simulink model "phantomx_sim_zero"  (R2025b)
settings: Solver=daessc  StartTime=0.0  StopTime=20  RelTol=1e-3
InitFcn:
  | % Parametri del filtro
  | num_filters = 18;       % Numero di filtri in parallelo (i tuoi 18 giunti/segnali)
  | tau = 0.05;             % Costante di tempo del filtro in secondi (modificabile)
  | a = 1 / tau;            % Polo del sistema
  | 
  | % 1. Creazione delle Matrici di Stato (State-Space)
  | % Matrice A (Dinamica del sistema): Diagonale con i poli
  | A = -a * eye(num_filters);
  | 
  | % Matrice B (Matrice di ingresso): Diagonale per mappare ogni input al suo stato
  | B = a * eye(num_filters);
  | 
  | % Matrice C (Matrice di uscita): Identità (vogliamo leggere gli stati direttamente)
  | C = eye(num_filters);
  | 
  | % Matrice D (Feedforward): Matrice di zeri (nessun collegamento diretto input-output)
  | D = zeros(num_filters, num_filters);
  | 
  | % 2. Creazione dell'oggetto State-Space in MATLAB
  | sys_filter = ss(A, B, C, D);
  | 
  | % Aggiungiamo i nomi per tenere tutto in ordine (opzionale ma consigliato)
  | sys_filter.InputName = strcat('Action_In_', string(1:num_filters));
  | sys_filter.OutputName = strcat('Filtered_Action_Out_', string(1:num_filters));
  | sys_filter.StateName = strcat('State_', string(1:num_filters));
  | 
  | % Mostra le proprietà del sistema creato
  | disp('Sistema State-Space creato con successo:');
  | sys_filter
  | 
  | run init_gait.m
undefined symbols (not defined in the file or in its folder): gait, X, Y, Z
libraries: sm_lib x298, nesl_utility x94, robotmaniplib x1
(part 5 of 5)

== system phantomx_sim_zero/tibia_lr ==
  Inertia : sm_lib/Body Elements/Inertia  InertiaType=Custom  Mass=0.024357719  MassUnits=kg  CenterOfMass=[0, 0, 0]  CenterOfMassUnits=m  MomentsOfInertia=[0.0051411124, 0.0081915737, 0.0011379812]  MomentsOfInertiaUnits=kg*m^2  ProductsOfInertia=[-1.9223094e-05, -2.4729049e-05, -0.0005753025500000001]  ProductsOfInertiaUnits=kg*m^2  GraphicType=None  MarkerShape=Inertia  MarkerSize=20  GraphicVisPropType=SimpleVisualProperties  GraphicDiffuseColor=[0.5 0.5 0.5]  GraphicOpacity=1  GraphicSpecularColor=[0.5 0.5 0.5 1.0]  GraphicAmbientColor=[0.15 0.15 0.15 1.0]  GraphicEmissiveColor=[0.0 0.0 0.0 1.0]  GraphicShininess=75
  InertiaOriginTransform : sm_lib/Frames and Transforms/Rigid Transform  RotationMethod=RotationSequence  FollAlignAxisA=+X  BaseAlignAxisA=+Y  FollAlignAxisB=+Y  BaseAlignAxisB=+Z  RotationStandardAxis=+Z  RotationAngle=0  RotationAngleUnits=deg  RotationArbitraryAxis=[0 0 1]  RotationSequenceAxes=BaseAxes  RotationSequence=XYZ  RotationSequenceAngles=[0, 0, 0]  RotationSequenceAnglesUnits=rad  RotationMatrix=[1 0 0;0 1 0;0 0 1]  Quaternion=[1 0 0 0]  TranslationMethod=Cartesian  TranslationCartesianOffset=[0, 0, 0]  TranslationCartesianOffsetUnits=m  TranslationStandardAxis=+Z  TranslationStandardOffset=0  TranslationStandardOffsetUnits=m  TranslationROffset=0  TranslationROffsetUnits=m  TranslationThetaOffset=0  TranslationThetaOffsetUnits=deg  TranslationZOffset=0  TranslationZOffsetUnits=m
  ReferenceFrame : sm_lib/Frames and Transforms/Reference Frame
  Visual : sm_lib/Body Elements/File Solid  ExtGeomFileName=phantomx_description-master/meshes/tibia_l.STL  UnitType=Custom  ExtGeomFileUnits=m  StepReaderType=HEX  ExportConvexHullGeometry=off  InertiaType=Custom  BasedOnType=DensityFromFile  Density=1000  DensityUnits=kg/m^3  Mass=0  MassUnits=kg  CenterOfMass=[0, 0, 0]  CenterOfMassUnits=m  MomentsOfInertia=[0, 0, 0]  MomentsOfInertiaUnits=kg*m^2  ProductsOfInertia=[0, 0, 0]  ProductsOfInertiaUnits=kg*m^2  GraphicType=FromGeometry  MarkerShape=Sphere  MarkerSize=10  GraphicVisPropType=SimpleVisualProperties  GraphicDiffuseColor=[0.2, 0.2, 0.2]  GraphicOpacity=1  GraphicSpecularColor=[0.5 0.5 0.5 1.0]  GraphicAmbientColor=[0.15 0.15 0.15 1.0]  GraphicEmissiveColor=[0.0 0.0 0.0 1.0]  GraphicShininess=75  DoExposeReferenceFrame=on  SerializedFrames=<Frames/>
  VisualOriginTransform : sm_lib/Frames and Transforms/Rigid Transform  RotationMethod=RotationSequence  FollAlignAxisA=+X  BaseAlignAxisA=+Y  FollAlignAxisB=+Y  BaseAlignAxisB=+Z  RotationStandardAxis=+Z  RotationAngle=0  RotationAngleUnits=deg  RotationArbitraryAxis=[0 0 1]  RotationSequenceAxes=BaseAxes  RotationSequence=XYZ  RotationSequenceAngles=[0, 0, 0]  RotationSequenceAnglesUnits=rad  RotationMatrix=[1 0 0;0 1 0;0 0 1]  Quaternion=[1 0 0 0]  TranslationMethod=Cartesian  TranslationCartesianOffset=[0, 0, 0]  TranslationCartesianOffsetUnits=m  TranslationStandardAxis=+Z  TranslationStandardOffset=0  TranslationStandardOffsetUnits=m  TranslationROffset=0  TranslationROffsetUnits=m  TranslationThetaOffset=0  TranslationThetaOffsetUnits=deg  TranslationZOffset=0  TranslationZOffsetUnits=m
  j_tibia_lr_AxisInvTransform : sm_lib/Frames and Transforms/Rigid Transform  RotationMethod=ArbitraryAxis  FollAlignAxisA=+X  BaseAlignAxisA=+Y  FollAlignAxisB=+Y  BaseAlignAxisB=+Z  RotationStandardAxis=+Z  RotationAngle=1.570796326794897  RotationAngleUnits=rad  RotationArbitraryAxis=[-0, 1, 0]  RotationSequenceAxes=FollowerAxes  RotationSequence=XYX  RotationSequenceAngles=[0 0 0]  RotationSequenceAnglesUnits=deg  RotationMatrix=[1 0 0;0 1 0;0 0 1]  Quaternion=[1 0 0 0]  TranslationMethod=Cartesian  TranslationCartesianOffset=[0, 0, 0]  TranslationCartesianOffsetUnits=m  TranslationStandardAxis=+Z  TranslationStandardOffset=0  TranslationStandardOffsetUnits=m  TranslationROffset=0  TranslationROffsetUnits=m  TranslationThetaOffset=0  TranslationThetaOffsetUnits=deg  TranslationZOffset=0  TranslationZOffsetUnits=m
  F : PMIOPort  Side=Left
  connections:
  Inertia/RConn1 -- InertiaOriginTransform/RConn1
  ReferenceFrame/RConn1 -- InertiaOriginTransform/LConn1 -- VisualOriginTransform/LConn1 -- j_tibia_lr_AxisInvTransform/LConn1
  Visual/RConn1 -- VisualOriginTransform/RConn1
  j_tibia_lr_AxisInvTransform/RConn1 -- F/RConn1

== system phantomx_sim_zero/tibia_rf ==
  Inertia : sm_lib/Body Elements/Inertia  InertiaType=Custom  Mass=0.024357719  MassUnits=kg  CenterOfMass=[0, 0, 0]  CenterOfMassUnits=m  MomentsOfInertia=[0.0051411124, 0.0081915737, 0.0011379812]  MomentsOfInertiaUnits=kg*m^2  ProductsOfInertia=[-1.9223094e-05, -2.4729049e-05, -0.0005753025500000001]  ProductsOfInertiaUnits=kg*m^2  GraphicType=None  MarkerShape=Inertia  MarkerSize=20  GraphicVisPropType=SimpleVisualProperties  GraphicDiffuseColor=[0.5 0.5 0.5]  GraphicOpacity=1  GraphicSpecularColor=[0.5 0.5 0.5 1.0]  GraphicAmbientColor=[0.15 0.15 0.15 1.0]  GraphicEmissiveColor=[0.0 0.0 0.0 1.0]  GraphicShininess=75
  InertiaOriginTransform : sm_lib/Frames and Transforms/Rigid Transform  RotationMethod=RotationSequence  FollAlignAxisA=+X  BaseAlignAxisA=+Y  FollAlignAxisB=+Y  BaseAlignAxisB=+Z  RotationStandardAxis=+Z  RotationAngle=0  RotationAngleUnits=deg  RotationArbitraryAxis=[0 0 1]  RotationSequenceAxes=BaseAxes  RotationSequence=XYZ  RotationSequenceAngles=[0, 0, 0]  RotationSequenceAnglesUnits=rad  RotationMatrix=[1 0 0;0 1 0;0 0 1]  Quaternion=[1 0 0 0]  TranslationMethod=Cartesian  TranslationCartesianOffset=[0, 0, 0]  TranslationCartesianOffsetUnits=m  TranslationStandardAxis=+Z  TranslationStandardOffset=0  TranslationStandardOffsetUnits=m  TranslationROffset=0  TranslationROffsetUnits=m  TranslationThetaOffset=0  TranslationThetaOffsetUnits=deg  TranslationZOffset=0  TranslationZOffsetUnits=m
  ReferenceFrame : sm_lib/Frames and Transforms/Reference Frame
  Visual : sm_lib/Body Elements/File Solid  ExtGeomFileName=phantomx_description-master/meshes/tibia_l.STL  UnitType=Custom  ExtGeomFileUnits=m  StepReaderType=HEX  ExportConvexHullGeometry=off  InertiaType=Custom  BasedOnType=DensityFromFile  Density=1000  DensityUnits=kg/m^3  Mass=0  MassUnits=kg  CenterOfMass=[0, 0, 0]  CenterOfMassUnits=m  MomentsOfInertia=[0, 0, 0]  MomentsOfInertiaUnits=kg*m^2  ProductsOfInertia=[0, 0, 0]  ProductsOfInertiaUnits=kg*m^2  GraphicType=FromGeometry  MarkerShape=Sphere  MarkerSize=10  GraphicVisPropType=SimpleVisualProperties  GraphicDiffuseColor=[0.2, 0.2, 0.2]  GraphicOpacity=1  GraphicSpecularColor=[0.5 0.5 0.5 1.0]  GraphicAmbientColor=[0.15 0.15 0.15 1.0]  GraphicEmissiveColor=[0.0 0.0 0.0 1.0]  GraphicShininess=75  DoExposeReferenceFrame=on  SerializedFrames=<Frames/>
  VisualOriginTransform : sm_lib/Frames and Transforms/Rigid Transform  RotationMethod=RotationSequence  FollAlignAxisA=+X  BaseAlignAxisA=+Y  FollAlignAxisB=+Y  BaseAlignAxisB=+Z  RotationStandardAxis=+Z  RotationAngle=0  RotationAngleUnits=deg  RotationArbitraryAxis=[0 0 1]  RotationSequenceAxes=BaseAxes  RotationSequence=XYZ  RotationSequenceAngles=[0, 0, 0]  RotationSequenceAnglesUnits=rad  RotationMatrix=[1 0 0;0 1 0;0 0 1]  Quaternion=[1 0 0 0]  TranslationMethod=Cartesian  TranslationCartesianOffset=[0, 0, 0]  TranslationCartesianOffsetUnits=m  TranslationStandardAxis=+Z  TranslationStandardOffset=0  TranslationStandardOffsetUnits=m  TranslationROffset=0  TranslationROffsetUnits=m  TranslationThetaOffset=0  TranslationThetaOffsetUnits=deg  TranslationZOffset=0  TranslationZOffsetUnits=m
  j_tibia_rf_AxisInvTransform : sm_lib/Frames and Transforms/Rigid Transform  RotationMethod=ArbitraryAxis  FollAlignAxisA=+X  BaseAlignAxisA=+Y  FollAlignAxisB=+Y  BaseAlignAxisB=+Z  RotationStandardAxis=+Z  RotationAngle=1.570796326794897  RotationAngleUnits=rad  RotationArbitraryAxis=[-0, 1, 0]  RotationSequenceAxes=FollowerAxes  RotationSequence=XYX  RotationSequenceAngles=[0 0 0]  RotationSequenceAnglesUnits=deg  RotationMatrix=[1 0 0;0 1 0;0 0 1]  Quaternion=[1 0 0 0]  TranslationMethod=Cartesian  TranslationCartesianOffset=[0, 0, 0]  TranslationCartesianOffsetUnits=m  TranslationStandardAxis=+Z  TranslationStandardOffset=0  TranslationStandardOffsetUnits=m  TranslationROffset=0  TranslationROffsetUnits=m  TranslationThetaOffset=0  TranslationThetaOffsetUnits=deg  TranslationZOffset=0  TranslationZOffsetUnits=m
  F : PMIOPort  Side=Left
  connections:
  Inertia/RConn1 -- InertiaOriginTransform/RConn1
  ReferenceFrame/RConn1 -- InertiaOriginTransform/LConn1 -- VisualOriginTransform/LConn1 -- j_tibia_rf_AxisInvTransform/LConn1
  Visual/RConn1 -- VisualOriginTransform/RConn1
  j_tibia_rf_AxisInvTransform/RConn1 -- F/RConn1

== system phantomx_sim_zero/tibia_rm ==
  Inertia : sm_lib/Body Elements/Inertia  InertiaType=Custom  Mass=0.024357719  MassUnits=kg  CenterOfMass=[0, 0, 0]  CenterOfMassUnits=m  MomentsOfInertia=[0.0051411124, 0.0081915737, 0.0011379812]  MomentsOfInertiaUnits=kg*m^2  ProductsOfInertia=[-1.9223094e-05, -2.4729049e-05, -0.0005753025500000001]  ProductsOfInertiaUnits=kg*m^2  GraphicType=None  MarkerShape=Inertia  MarkerSize=20  GraphicVisPropType=SimpleVisualProperties  GraphicDiffuseColor=[0.5 0.5 0.5]  GraphicOpacity=1  GraphicSpecularColor=[0.5 0.5 0.5 1.0]  GraphicAmbientColor=[0.15 0.15 0.15 1.0]  GraphicEmissiveColor=[0.0 0.0 0.0 1.0]  GraphicShininess=75
  InertiaOriginTransform : sm_lib/Frames and Transforms/Rigid Transform  RotationMethod=RotationSequence  FollAlignAxisA=+X  BaseAlignAxisA=+Y  FollAlignAxisB=+Y  BaseAlignAxisB=+Z  RotationStandardAxis=+Z  RotationAngle=0  RotationAngleUnits=deg  RotationArbitraryAxis=[0 0 1]  RotationSequenceAxes=BaseAxes  RotationSequence=XYZ  RotationSequenceAngles=[0, 0, 0]  RotationSequenceAnglesUnits=rad  RotationMatrix=[1 0 0;0 1 0;0 0 1]  Quaternion=[1 0 0 0]  TranslationMethod=Cartesian  TranslationCartesianOffset=[0, 0, 0]  TranslationCartesianOffsetUnits=m  TranslationStandardAxis=+Z  TranslationStandardOffset=0  TranslationStandardOffsetUnits=m  TranslationROffset=0  TranslationROffsetUnits=m  TranslationThetaOffset=0  TranslationThetaOffsetUnits=deg  TranslationZOffset=0  TranslationZOffsetUnits=m
  ReferenceFrame : sm_lib/Frames and Transforms/Reference Frame
  Visual : sm_lib/Body Elements/File Solid  ExtGeomFileName=phantomx_description-master/meshes/tibia_l.STL  UnitType=Custom  ExtGeomFileUnits=m  StepReaderType=HEX  ExportConvexHullGeometry=off  InertiaType=Custom  BasedOnType=DensityFromFile  Density=1000  DensityUnits=kg/m^3  Mass=0  MassUnits=kg  CenterOfMass=[0, 0, 0]  CenterOfMassUnits=m  MomentsOfInertia=[0, 0, 0]  MomentsOfInertiaUnits=kg*m^2  ProductsOfInertia=[0, 0, 0]  ProductsOfInertiaUnits=kg*m^2  GraphicType=FromGeometry  MarkerShape=Sphere  MarkerSize=10  GraphicVisPropType=SimpleVisualProperties  GraphicDiffuseColor=[0.2, 0.2, 0.2]  GraphicOpacity=1  GraphicSpecularColor=[0.5 0.5 0.5 1.0]  GraphicAmbientColor=[0.15 0.15 0.15 1.0]  GraphicEmissiveColor=[0.0 0.0 0.0 1.0]  GraphicShininess=75  DoExposeReferenceFrame=on  SerializedFrames=<Frames/>
  VisualOriginTransform : sm_lib/Frames and Transforms/Rigid Transform  RotationMethod=RotationSequence  FollAlignAxisA=+X  BaseAlignAxisA=+Y  FollAlignAxisB=+Y  BaseAlignAxisB=+Z  RotationStandardAxis=+Z  RotationAngle=0  RotationAngleUnits=deg  RotationArbitraryAxis=[0 0 1]  RotationSequenceAxes=BaseAxes  RotationSequence=XYZ  RotationSequenceAngles=[0, 0, 0]  RotationSequenceAnglesUnits=rad  RotationMatrix=[1 0 0;0 1 0;0 0 1]  Quaternion=[1 0 0 0]  TranslationMethod=Cartesian  TranslationCartesianOffset=[0, 0, 0]  TranslationCartesianOffsetUnits=m  TranslationStandardAxis=+Z  TranslationStandardOffset=0  TranslationStandardOffsetUnits=m  TranslationROffset=0  TranslationROffsetUnits=m  TranslationThetaOffset=0  TranslationThetaOffsetUnits=deg  TranslationZOffset=0  TranslationZOffsetUnits=m
  j_tibia_rm_AxisInvTransform : sm_lib/Frames and Transforms/Rigid Transform  RotationMethod=ArbitraryAxis  FollAlignAxisA=+X  BaseAlignAxisA=+Y  FollAlignAxisB=+Y  BaseAlignAxisB=+Z  RotationStandardAxis=+Z  RotationAngle=1.570796326794897  RotationAngleUnits=rad  RotationArbitraryAxis=[-0, 1, 0]  RotationSequenceAxes=FollowerAxes  RotationSequence=XYX  RotationSequenceAngles=[0 0 0]  RotationSequenceAnglesUnits=deg  RotationMatrix=[1 0 0;0 1 0;0 0 1]  Quaternion=[1 0 0 0]  TranslationMethod=Cartesian  TranslationCartesianOffset=[0, 0, 0]  TranslationCartesianOffsetUnits=m  TranslationStandardAxis=+Z  TranslationStandardOffset=0  TranslationStandardOffsetUnits=m  TranslationROffset=0  TranslationROffsetUnits=m  TranslationThetaOffset=0  TranslationThetaOffsetUnits=deg  TranslationZOffset=0  TranslationZOffsetUnits=m
  F : PMIOPort  Side=Left
  connections:
  Inertia/RConn1 -- InertiaOriginTransform/RConn1
  ReferenceFrame/RConn1 -- InertiaOriginTransform/LConn1 -- VisualOriginTransform/LConn1 -- j_tibia_rm_AxisInvTransform/LConn1
  Visual/RConn1 -- VisualOriginTransform/RConn1
  j_tibia_rm_AxisInvTransform/RConn1 -- F/RConn1

== system phantomx_sim_zero/tibia_rr ==
  Inertia : sm_lib/Body Elements/Inertia  InertiaType=Custom  Mass=0.024357719  MassUnits=kg  CenterOfMass=[0, 0, 0]  CenterOfMassUnits=m  MomentsOfInertia=[0.0051411124, 0.0081915737, 0.0011379812]  MomentsOfInertiaUnits=kg*m^2  ProductsOfInertia=[-1.9223094e-05, -2.4729049e-05, -0.0005753025500000001]  ProductsOfInertiaUnits=kg*m^2  GraphicType=None  MarkerShape=Inertia  MarkerSize=20  GraphicVisPropType=SimpleVisualProperties  GraphicDiffuseColor=[0.5 0.5 0.5]  GraphicOpacity=1  GraphicSpecularColor=[0.5 0.5 0.5 1.0]  GraphicAmbientColor=[0.15 0.15 0.15 1.0]  GraphicEmissiveColor=[0.0 0.0 0.0 1.0]  GraphicShininess=75
  InertiaOriginTransform : sm_lib/Frames and Transforms/Rigid Transform  RotationMethod=RotationSequence  FollAlignAxisA=+X  BaseAlignAxisA=+Y  FollAlignAxisB=+Y  BaseAlignAxisB=+Z  RotationStandardAxis=+Z  RotationAngle=0  RotationAngleUnits=deg  RotationArbitraryAxis=[0 0 1]  RotationSequenceAxes=BaseAxes  RotationSequence=XYZ  RotationSequenceAngles=[0, 0, 0]  RotationSequenceAnglesUnits=rad  RotationMatrix=[1 0 0;0 1 0;0 0 1]  Quaternion=[1 0 0 0]  TranslationMethod=Cartesian  TranslationCartesianOffset=[0, 0, 0]  TranslationCartesianOffsetUnits=m  TranslationStandardAxis=+Z  TranslationStandardOffset=0  TranslationStandardOffsetUnits=m  TranslationROffset=0  TranslationROffsetUnits=m  TranslationThetaOffset=0  TranslationThetaOffsetUnits=deg  TranslationZOffset=0  TranslationZOffsetUnits=m
  ReferenceFrame : sm_lib/Frames and Transforms/Reference Frame
  Visual : sm_lib/Body Elements/File Solid  ExtGeomFileName=phantomx_description-master/meshes/tibia_l.STL  UnitType=Custom  ExtGeomFileUnits=m  StepReaderType=HEX  ExportConvexHullGeometry=off  InertiaType=Custom  BasedOnType=DensityFromFile  Density=1000  DensityUnits=kg/m^3  Mass=0  MassUnits=kg  CenterOfMass=[0, 0, 0]  CenterOfMassUnits=m  MomentsOfInertia=[0, 0, 0]  MomentsOfInertiaUnits=kg*m^2  ProductsOfInertia=[0, 0, 0]  ProductsOfInertiaUnits=kg*m^2  GraphicType=FromGeometry  MarkerShape=Sphere  MarkerSize=10  GraphicVisPropType=SimpleVisualProperties  GraphicDiffuseColor=[0.2, 0.2, 0.2]  GraphicOpacity=1  GraphicSpecularColor=[0.5 0.5 0.5 1.0]  GraphicAmbientColor=[0.15 0.15 0.15 1.0]  GraphicEmissiveColor=[0.0 0.0 0.0 1.0]  GraphicShininess=75  DoExposeReferenceFrame=on  SerializedFrames=<Frames/>
  VisualOriginTransform : sm_lib/Frames and Transforms/Rigid Transform  RotationMethod=RotationSequence  FollAlignAxisA=+X  BaseAlignAxisA=+Y  FollAlignAxisB=+Y  BaseAlignAxisB=+Z  RotationStandardAxis=+Z  RotationAngle=0  RotationAngleUnits=deg  RotationArbitraryAxis=[0 0 1]  RotationSequenceAxes=BaseAxes  RotationSequence=XYZ  RotationSequenceAngles=[0, 0, 0]  RotationSequenceAnglesUnits=rad  RotationMatrix=[1 0 0;0 1 0;0 0 1]  Quaternion=[1 0 0 0]  TranslationMethod=Cartesian  TranslationCartesianOffset=[0, 0, 0]  TranslationCartesianOffsetUnits=m  TranslationStandardAxis=+Z  TranslationStandardOffset=0  TranslationStandardOffsetUnits=m  TranslationROffset=0  TranslationROffsetUnits=m  TranslationThetaOffset=0  TranslationThetaOffsetUnits=deg  TranslationZOffset=0  TranslationZOffsetUnits=m
  j_tibia_rr_AxisInvTransform : sm_lib/Frames and Transforms/Rigid Transform  RotationMethod=ArbitraryAxis  FollAlignAxisA=+X  BaseAlignAxisA=+Y  FollAlignAxisB=+Y  BaseAlignAxisB=+Z  RotationStandardAxis=+Z  RotationAngle=1.570796326794897  RotationAngleUnits=rad  RotationArbitraryAxis=[-0, 1, 0]  RotationSequenceAxes=FollowerAxes  RotationSequence=XYX  RotationSequenceAngles=[0 0 0]  RotationSequenceAnglesUnits=deg  RotationMatrix=[1 0 0;0 1 0;0 0 1]  Quaternion=[1 0 0 0]  TranslationMethod=Cartesian  TranslationCartesianOffset=[0, 0, 0]  TranslationCartesianOffsetUnits=m  TranslationStandardAxis=+Z  TranslationStandardOffset=0  TranslationStandardOffsetUnits=m  TranslationROffset=0  TranslationROffsetUnits=m  TranslationThetaOffset=0  TranslationThetaOffsetUnits=deg  TranslationZOffset=0  TranslationZOffsetUnits=m
  F : PMIOPort  Side=Left
  connections:
  Inertia/RConn1 -- InertiaOriginTransform/RConn1
  ReferenceFrame/RConn1 -- InertiaOriginTransform/LConn1 -- VisualOriginTransform/LConn1 -- j_tibia_rr_AxisInvTransform/LConn1
  Visual/RConn1 -- VisualOriginTransform/RConn1
  j_tibia_rr_AxisInvTransform/RConn1 -- F/RConn1

== matlab function phantomx_sim_zero/MATLAB Function1 ==
  data: x output; t_in input; y output; z output; T input; S input; H input; z0 input; duty input
function [x, y, z] = tripod_gait(t_in, T, S, H, z0, duty)
%#codegen
    [x, y, z] = tripod_trajectory(t_in, T, S, H, z0, duty);
end

== matlab function phantomx_sim_zero/MATLAB Function2 ==
  settings: updateMethod=DISCRETE
  data: z input; z_lf output; c_lf input; c_lr input; c_rm input; z_lr output; z_rm output; t input
function [z_lf, z_lr, z_rm] = fcn(z, c_lf, c_lr, c_rm, t)

z_nominal  = 0.14;   
v_search   = 0.06; 
z_ext_max  = 0.03;    

persistent z_hold_lf z_hold_lr z_hold_rm
persistent z_ext_lf  z_ext_lr  z_ext_rm
persistent t_prev

if isempty(z_hold_lf) || t < 0.5
    z_hold_lf = z;
    z_hold_lr = z;
    z_hold_rm = z;
    
    z_ext_lf  = 0;
    z_ext_lr  = 0;
    z_ext_rm  = 0;
    
    t_prev    = t;
end

dt = t - t_prev;
if dt <= 0 || dt > 0.1
    dt = 0.001; 
end
t_prev = t;

if c_lf == 0
    if z >= (z_nominal - 0.002)
        z_ext_lf  = min(z_ext_lf + v_search * dt, z_ext_max);
        z_hold_lf = z + z_ext_lf;
        z_lf      = z_hold_lf;
    else
        z_ext_lf  = 0;
        z_hold_lf = z;
        z_lf      = z;
    end
else
    z_lf = min(z + z_ext_lf, z_hold_lf);
end


if c_lr == 0
    if z >= (z_nominal - 0.002)
        z_ext_lr  = min(z_ext_lr + v_search * dt, z_ext_max);
        z_hold_lr = z + z_ext_lr;
        z_lr      = z_hold_lr;
    else
        z_ext_lr  = 0;
        z_hold_lr = z;
        z_lr      = z;
    end
else
    z_lr = min(z + z_ext_lr, z_hold_lr);
end


if c_rm == 0
    if z >= (z_nominal - 0.002)
        z_ext_rm  = min(z_ext_rm + v_search * dt, z_ext_max);
        z_hold_rm = z + z_ext_rm;
        z_rm      = z_hold_rm;
    else
        z_ext_rm  = 0;
        z_hold_rm = z;
        z_rm      = z;
    end
else
    z_rm = min(z + z_ext_rm, z_hold_rm);
end

== matlab function phantomx_sim_zero/MATLAB Function3 ==
  settings: updateMethod=DISCRETE
  data: z input; z_rf output; c_rf input; c_rr input; c_lm input; z_rr output; z_lm output; t input
function [z_rf, z_rr, z_lm] = fcn(z, c_rf, c_rr, c_lm, t)

z_nominal  = 0.14; 
v_search   = 0.06;
z_ext_max  = 0.03;  

persistent z_hold_rf z_hold_rr z_hold_lm
persistent z_ext_rf  z_ext_rr  z_ext_lm
persistent t_prev

if isempty(z_hold_rf) || t < 0.5
    z_hold_rf = z;
    z_hold_rr = z;
    z_hold_lm = z;
    
    z_ext_rf  = 0;
    z_ext_rr  = 0;
    z_ext_lm  = 0;
    
    t_prev    = t;
end

dt = t - t_prev;
if dt <= 0 || dt > 0.1
    dt = 0.001; 
end
t_prev = t;


if c_rf == 0
    if z >= (z_nominal - 0.002)
        z_ext_rf  = min(z_ext_rf + v_search * dt, z_ext_max);
        z_hold_rf = z + z_ext_rf;
        z_rf      = z_hold_rf;
    else
        z_ext_rf  = 0;
        z_hold_rf = z;
        z_rf      = z;
    end
else
    z_rf = min(z + z_ext_rf, z_hold_rf);
end

if c_rr == 0
    if z >= (z_nominal - 0.002)
        z_ext_rr  = min(z_ext_rr + v_search * dt, z_ext_max);
        z_hold_rr = z + z_ext_rr;
        z_rr      = z_hold_rr;
    else
        z_ext_rr  = 0;
        z_hold_rr = z;
        z_rr      = z;
    end
else
    z_rr = min(z + z_ext_rr, z_hold_rr);
end


if c_lm == 0
    if z >= (z_nominal - 0.002)
        z_ext_lm  = min(z_ext_lm + v_search * dt, z_ext_max);
        z_hold_lm = z + z_ext_lm;
        z_lm      = z_hold_lm;
    else
        z_ext_lm  = 0;
        z_hold_lm = z;
        z_lm      = z;
    end
else
    z_lm = min(z + z_ext_lm, z_hold_lm);
end

== matlab function phantomx_sim_zero/MR ==
  data: x input; theta output; y input; z input; phi output; psi output; side input; alpha input
function [theta, phi, psi] = leg_ik(x, y, z, side, alpha)
    [theta, phi, psi] = inv_kyn(x, y, z, side, alpha);
end

== matlab function phantomx_sim_zero/RR ==
  data: x input; theta output; y input; z input; phi output; psi output; side input; alpha input
function [theta, phi, psi] = leg_ik(x, y, z, side, alpha)
    [theta, phi, psi] = inv_kyn(x, y, z, side, alpha);
end

== matlab function phantomx_sim_zero/FR ==
  data: x input; theta output; y input; z input; phi output; psi output; side input; alpha input
function [theta, phi, psi] = leg_ik(x, y, z, side, alpha)
    [theta, phi, psi] = inv_kyn(x, y, z, side, alpha);
end

== matlab function phantomx_sim_zero/RL ==
  data: x input; theta output; y input; z input; phi output; psi output; side input; alpha input
function [theta, phi, psi] = leg_ik(x, y, z, side, alpha)
    [theta, phi, psi] = inv_kyn(x, y, z, side, alpha);
end

== matlab function phantomx_sim_zero/ML ==
  data: x input; theta output; y input; z input; phi output; psi output; side input; alpha input
function [theta, phi, psi] = leg_ik(x, y, z, side, alpha)
    [theta, phi, psi] = inv_kyn(x, y, z, side, alpha);
end

== matlab function phantomx_sim_zero/FL ==
  data: x input; theta output; y input; z input; phi output; psi output; side input; alpha input
function [theta, phi, psi] = leg_ik(x, y, z, side, alpha)
    [theta, phi, psi] = inv_kyn(x, y, z, side, alpha);
end

== matlab function phantomx_sim_zero/MATLAB Function ==
  data: x output; t_in input; y output; z output; T input; S input; H input; z0 input; duty input
function [x, y, z] = tripod_gait(t_in, T, S, H, z0, duty)
%#codegen
    [x, y, z] = tripod_trajectory(t_in, T, S, H, z0, duty);
end
